simulink library "SUB_ECU_L4_MABX_HW_Interface_PIC_PB"  (R2018a)
settings: Solver=VariableStepAuto  StartTime=0.0  StopTime=10.0  RelTol=1e-3
PostLoadFcn:
  | , if any(exist('dsrtsu_mdlpostloadfcn', 'file') == [2, 3, 6]), try dsrtsu_mdlpostloadfcn('Execute', bdroot); catch fprintf('Error in PostLoadFcn (dsrtsu_mdlpostloadfcn) for model "%s":\n %s\n', bdroot, lasterr); end, end,
undefined symbols (not defined in the file or in its folder): CANR_PROPB_REAX_3_13_CHANNEL_APV, CANR_PROPB_REAX_4_13_CHANNEL_APV, CANR_PROPB_XPR_1_50_CHANNEL_APV, ENUM_CAN_RX_T, ENUM_CAN_TX_T, ENUM_REAX_OPERATION_MODE_T, ENUM_SIGNAL_HEALTH_T, ENUM_XBR_CONTROL_MODE_T, ENUM_XBR_EBI_MODE_T, ENUM_XBR_PASS_THROUGH_ACTIVE_T, ENUM_XBR_PRIORITY_T, ENUM_XPR_INHIBIT_PARK_MANUAL_T, ENUM_XPR_INHIBIT_UNPARK_MANUAL_T, ENUM_XPR_PARK_MANUAL_T, ENUM_XPR_UNPARK_MANUAL_T, PROPB_REAX_1_E4_DES_POS_SIG_SRC_APV, PROPB_REAX_1_E4_DESIRED_OPMODE_APV, PROPB_REAX_1_E4_DESIRED_POSITION_APV, PROPB_REAX_CHANNEL_APV, ptc_matlab_lib
libraries: PTC_MBDS_LIB x293, rtican x158, simulink x61, EmE_MBD_Blockset x38, rti1401lib_dio_type4 x14, simulink_need_slupdate x7, $bdroot x5, rti1401lib_adc_type4 x3, rtmapslib x3, dsa_tcpip_lib x2, SUB_ECU_L4_MABX_HW_Interface_PTC_1571 x1, rtitasklib x1
(part 27 of 49)

== system SUB_ECU_L4_MABX_HW_Interface_PIC_PB/CAN_Out_PIC_PB/CAN_TX_20ms/CAN_TX_STD_ODOMETRY/TX_CAN6 ==
  Enable : Inport
  Data : Inport  Port=2
  Bus Selector4 : BusSelector  OutputSignals=INPUTS.CAN.EBC2_0B.FrontAxleSpeed,INPUTS.CAN.VDC2_0B.SPN1807_SteeringWheelAngle,INPUTS.CAN.VDC2_0B.SPN1808_YawRate,INPUTS.CAN.VDC2_0B.SPN1810_LongitudinalAcceleration
  Data Type Conversion{,1..3} (4 alike) : DataTypeConversion  OutDataTypeStr=double
  Std_OdometryData : rtican/RTICAN Transmit (TX)   Reserved1=[]  Reserved2=[]  Reserved3=[]  Reserved4=[]  SfcnMessage=[]  Msg_Struct=[]  BoardTypeNo=[]  BoardNo=[]  ChannelNo=[]  Parameters=[]  DialogFcn=[]  UnitName=[]  Revision=[]  UnitValues=[]  DSProperties=struct('RTI',struct('Version',uint32(5),'BlockType',struct('isSLSource',uint8(1),'isSLSink',uint8(1),'isHWSource',uint8(0),'isHWSink',uint8(0),'isSetup',uint8(0),'isInline',uint8(1),'isNonInline',uint8(0),'isInterrupt',uint8(0),'isChannelwise',uint8(0)),'IOBoardType','RTICAN','UnitType','MESSAGE','Identifier','TX','DialogType','MSVC','BlockSet','RTICAN','SlaveProcessor','CAN'))  RTIBlockInterface=struct('InputPortsWidth',int32([1 1 1 1]),'InputPortsActive',[1 1 1 1],'InputPortsName',{{'SPN904_FrontAxleSpeed','SPN1807_SteeringWheelAngle','SPN1808_YawRate','SPN1810_LongitudinalAcceleration'}},'InputPortsDataType',{{'SS_DOUBLE','SS_DOUBLE','SS_DOUBLE','SS_DOUBLE'}},'OutputPortsWidth',int32([1 1 1 1]),'OutputPortsActive',[1 1 1 1],'OutputPortsName',{{['TX status'],['TX time'],['TX delta time'],['TX delay time']}},'DialogFcn','rtican_message_interface_gui','BlockDisplay',{{'','center'}},'IconTransparency','on','InitLevel',3,'BlockName',struct('Token',{{'Std_OdometryData'}}),'SampleTime',{{-1}},'TriggerPort',{{'none'}},'EnablePort',{{'yes'}})  RTIBlockParameters="struct('BoardTypeNo',{{1,'OFF',[]}},'BoardNo',{{3,'ON',[1 16]}},'ChannelNo',{{2,'ON',[1 2]}},'Parameters',{{struct('DataFileSupport',struct('DataFileSelectedMaster',1,'DataFileSelectedLocal',0,'DataFileName',['c:\\users\\gavin.coelho\\repos\\l4 svn\\branches\\gennaro\\project_l4\\src\\projectlibrary\\dbc\\mabx_can6_beta4.dbc|c:\\users\\gavin.coelho\\repos\\l4 svn\\branches\\gennaro\\project_l4\\src\\candb\\mabx_can4_chrisbalton.dbc|'],'DataFileDate',{{{['10-Feb-2017 15:17:28']}}},'SelectedFile',['<no file selected>']),'Options',struct('StatusSelected',1,'TimeSelected',1,'DeltaTimeSelected',1,'DelayTimeSelected',1,'DelayTimeTXCommandSelected',0,'EncodeSetUnusedBitsToOne',1,'EnableMsgLoopback',0,'TriggerPort',struct('Selected',0,'TriggerType',0),'EnablePortSelected',1,'SignalOnPortnameSelected',1,'UserCoding',struct('Selected',0,'InterfaceFile','UserEncodingFile','FcnName','UserEncodeFcn','InportSelected',0,'InportWidth',1,'OutportSelected',0,'OutportWidth',1),'TerminationMsg',struct('Selected',0,'Byte0_7','0'),'InitialMsg',struct('Selected',0,'Byte0_7','0')),'Message',struct('MsgOnBlocknameSelected',1,'MsgName','Std_OdometryData','MsgIdFormat',0,'MsgId',10,'MsgLength',8,'NumSignals',4,'SampleTime',-1,'StartTime',struct('Selected',0,'Value',0),'AutoRepeatTime',struct('Selected',0,'Value',0.1),'Timeout',struct('Selected',0,'Value',0.1),'DelayTime',struct('Selected',0,'Value',0.1),'Signal',struct('SgnName',{'SPN904_FrontAxleSpeed','SPN1807_SteeringWheelAngle','SPN1808_YawRate','SPN1810_LongitudinalAcceleration'},'SgnStartBit',{0,16,32,48},'SgnLength',{16,16,16,8},'SgnType',{0,0,0,0},'ModeValue',{-1,-1,-1,-1},'DataType',{0,0,0,0},'ByteLayout',{0,0,0,0},'Factor',{2^-8,2^-10,2^-13,0.1},'Offset',{0,-31.374,-3.92,-12.5},'SgnComment',{{['The average speed of the two front wheels.']},{['The main operator`s steering wheel angle (on the steering column, not the actual wheel angle).']},{['Indicates the rate of rotation about the vertical axis (i.e. the z-axis).  A positive yaw rate signal results when the vehicle turns counter-clockwise.']},{['Indicates the longitudinal acceleration of the vehicle. A positive longitudinal acceleration signal results when the vehicle speed increases, regardless of driving the vehicle forward or backward.']}},'SgnUnit',{'km/h','rad','rad/s','m/s^2'},'Min',{0,0,0,0},'Max',{0,0,0,0},'SLDataType',{'SS_DOUBLE','SS_DOUBLE','SS_DOUBLE','SS_DOUBLE'}),'MsgIdNumFormat',1,'MsgComment',{{''}}),'Version',1.2,'general',struct('isFromLib',0)),'OFF',[]}},'GroupId',{{struct('Group',{{'RTICAN'}},'No',6,'Behavior',{{'NAMECHANGE'}},'BlockType',{{'SINK'}},'NameChangeFlag',0),'OFF',[]}},'SFcnRTICANMessage',{{struct('MsgType','TX','SFcnPortType','Scalar','MsgName','Std_OdometryData','MsgIdFormat','STD','MsgId',10,'MsgLength',8,'NumSignals',4,'SampleTime',-1,'StartTime',struct('Selected','no','Value',0),'AutoRepeatTime',struct('Selected','no','Value',0.1),'Timeout',struct('Selected','no','Value',0.1),'Signal',struct('SgnName',{'SPN904_FrontAxleSpeed','SPN1807_SteeringWheelAngle','SPN1808_YawRate','SPN1810_LongitudinalAcceleration'},'SgnStartBit',{0,16,32,48},'SgnLength',{16,16,16,8},'SgnType',{'standard','standard','standard','standard'},'ModeValue',{-1,-1,-1,-1},'DataType',{['unsigned int'],['unsigned int'],['unsigned int'],['unsigned int']},'ByteLayout',{['little endian'],['little endian'],['little endian'],['little endian']},'Factor',{2^-8,2^-10,2^-13,0.1},'Offset',{0,-31.374,-3.92,-12.5},'SLDataType',{'SS_DOUBLE','SS_DOUBLE','SS_DOUBLE','SS_DOUBLE'}),'StatusSelected','yes','TimeSelected','yes','DeltaTimeSelected','yes','DelayTimeSelected','yes','DelayTimeTXCommandSelected','no','EncodeSetUnusedBitsToOne','yes','EnableMsgLoopback','no','TriggerPort',struct('Selected','no','TriggerType',0),'EnablePortSelected','yes','UserCoding',struct('Selected','no','InterfaceFile','UserEncodingFile','FcnName','UserEncodeFcn','InportSelected','no','InportWidth',1,'OutportSelected','no','OutportWidth',1),'TerminationMsg',struct('Selected','no','Byte0','0x00','Byte1','0x00','Byte2','0x00','Byte3','0x00','Byte4','0x00','Byte5','0x00','Byte6','0x00','Byte7','0x00'),'InitialMsg',struct('Selected','no','Byte0','0x00','Byte1','0x00','Byte2','0x00','Byte3','0x00','Byte4','0x00','Byte5','0x00','Byte6','0x00','Byte7','0x00'),'BoardType','DS1','BoardNo',3,'ControllerNo',2),'OFF',[]}},'TLCFileName',{{'rtican_tx_message','OFF',[]}})"  RTISFcnParameters=struct('SFcnRTICANMessage','struct','TLCFileName','char')  RTIBlockParaDefault=struct('BoardTypeNo',4302,'BoardNo',1,'ChannelNo',1,'Parameters',struct('DataFileSupport',struct('DataFileSelectedMaster',0,'DataFileSelectedLocal',0,'DataFileName','','DataFileDate','','SelectedFile',['<no file selected>']),'Options',struct('StatusSelected',1,'TimeSelected',1,'DeltaTimeSelected',1,'DelayTimeSelected',1,'DelayTimeTXCommandSelected',0,'EncodeSetUnusedBitsToOne',0,'EnableMsgLoopback',0,'TriggerPort',struct('Selected',0,'TriggerType','rising'),'EnablePortSelected',0,'SignalOnPortnameSelected',1,'UserCoding',struct('Selected',0,'InterfaceFile','UserEncodingFile','FcnName','UserEncodeFcn','InportSelected',0,'InportWidth',1,'OutportSelected',0,'OutportWidth',1),'TerminationMsg',struct('Selected',0,'Byte0_7','0'),'InitialMsg',struct('Selected',0,'Byte0_7','0')),'Message',struct('MsgOnBlocknameSelected',0,'MsgName',['TX Message'],'MsgIdFormat',0,'MsgId',100,'MsgLength',8,'NumSignals',1,'SampleTime',-1,'StartTime',struct('Selected',0,'Value',0),'AutoRepeatTime',struct('Selected',0,'Value',0.1),'Timeout',struct('Selected',0,'Value',0.1),'DelayTime',struct('Selected',0,'Value',0.1),'Signal',struct('SgnName',['TX signal'],'SgnStartBit',0,'SgnLength',8,'SgnType',0,'ModeValue',-1,'DataType',0,'SLDataType','SS_DOUBLE','ByteLayout',0,'Factor',1,'Offset',0,'Min',0,'Max',255,'SgnComment',{{}},'SgnUnit',''),'MsgIdNumFormat',0,'MsgComment',{{''}}),'Version',1.2,'general',struct('isFromLib',1)),'GroupId',struct('Group',{{'RTICAN'}},'No',1,'Behavior',{{'NAMECHANGE'}},'BlockType',{{'SINK'}},'NameChangeFlag',0),'SFcnRTICANMessage',struct('MsgType','TX','MsgName',['TX Message'],'MsgIdFormat','STD','MsgId',100,'MsgLength',2,'NumSignals',1,'SampleTime',-1,'StartTime',struct('Selected','no','Value',0),'AutoRepeatTime',struct('Selected','no','Value',0.1),'Timeout',struct('Selected','no','Value',0.1),'DelayTime',struct('Selected','no','Value',0.1),'Signal',struct('SgnName',['TX signal'],'SgnStartBit',0,'SgnLength',8,'SgnType','standard','ModeValue',-1,'DataType',['unsigned int'],'ByteLayout',['little endian'],'SLDataType','SS_DOUBLE','Factor',1,'Offset',0),'StatusSelected','yes','TimeSelected','yes','DeltaTimeSelected','yes','DelayTimeSelected','yes','EnablePortSelected','no','EnableMsgLoopback','no','DelayTimeTXCommandSelected','no','EncodeSetUnusedBitsToOne','no','UserCoding',struct('Selected','no','InterfaceFile','UserDecodingFile','FcnName','UserDecodeFcn','InportSelected','no','InportWidth',1,'OutportSelected','no','OutportWidth',1),'TerminationMsg',struct('Selected','no','Byte0','0x00','Byte1','0x00','Byte2','0x00','Byte3','0x00','Byte4','0x00','Byte5','0x00','Byte6','0x00','Byte7','0x00'),'InitialMsg',struct('Selected','no','Byte0','0x00','Byte1','0x00','Byte2','0x00','Byte3','0x00','Byte4','0x00','Byte5','0x00','Byte6','0x00','Byte7','0x00'),'TriggerPort',struct('Selected','no','TriggerType','rising'),'BoardType','DS4302','BoardNo',1,'ControllerNo',1,'SFcnPortType','Scalar'),'TLCFileName','rtican_tx_message')
      settings: AttributesFormatString=Group Id: RTICAN6\n  SourceProductName=dSPACE RTI CAN Blockset
  Terminator{,1..3} (4 alike) : Terminator
      settings: InitFcn=|
      | try
      |    MBDS_BlockCallback('Update', gcb);
      | end
  wires:
  Data Type Conversion3/1 -> Std_OdometryData/4
  Data Type Conversion2/1 -> Std_OdometryData/3
  Data Type Conversion1/1 -> Std_OdometryData/2
  Data Type Conversion/1 -> Std_OdometryData/1
  Data/1 -> Bus Selector4/1
  Std_OdometryData/1 -> Terminator/1
  Std_OdometryData/3 -> Terminator2/1
  Std_OdometryData/4 -> Terminator3/1
  Std_OdometryData/2 -> Terminator1/1
  Enable/1 -> Std_OdometryData/Enable
  Bus Selector4/3 -> Data Type Conversion2/1  "<SPN1808_YawRate>"
  Bus Selector4/2 -> Data Type Conversion1/1  "<SPN1807_SteeringWheelAngle>"
  Bus Selector4/4 -> Data Type Conversion3/1  "<SPN1810_LongitudinalAcceleration>"
  Bus Selector4/1 -> Data Type Conversion/1  "<FrontAxleSpeed>"

== system SUB_ECU_L4_MABX_HW_Interface_PIC_PB/CAN_Out_PIC_PB/CAN_TX_20ms/Encode_PropB_2C2_XPR/CAN_ID_PropB_2C2_XPR_65 ==
  note: 0xCFF5665
  Bitwise Operator17 : simulink/Logic and Bit Operations/Bitwise Operator  logicop=OR  UseBitMask=off  NumInputPorts=6  BitMask=bin2dec('11011001')  BitMaskRealWorld=Stored Integer
  Data Type Conversion{6..11} (6 alike) : DataTypeConversion  OutDataTypeStr=uint32
  DataPage : Constant  Value=boolean(0)
  ExtendedDataPage : Constant  Value=boolean(0)
  PDUFormat : Constant  Value=uint8(hex2dec('FF'))
  PDUSpecific : Constant  Value=uint8(hex2dec('56'))
  Priority : Constant  Value=uint8(3)
  Shift_Arithmetic 5 : ArithShift  BitShiftNumber=-26
  Shift_Arithmetic 6 : ArithShift  BitShiftNumber=-25
  Shift_Arithmetic 7 : ArithShift  BitShiftNumber=-24
  Shift_Arithmetic 8 : ArithShift  BitShiftNumber=-16
  Shift_Arithmetic 9 : ArithShift  BitShiftNumber=-8
  SourceAddress : Constant  Value=uint8(hex2dec('65'))
  MessageID : Outport
  wires:
  Bitwise Operator17/1 -> MessageID/1
  Data Type Conversion11/1 -> Bitwise Operator17/6
  Data Type Conversion10/1 -> Shift_Arithmetic 9/1
  Data Type Conversion9/1 -> Shift_Arithmetic 8/1
  Data Type Conversion8/1 -> Shift_Arithmetic 7/1
  Data Type Conversion7/1 -> Shift_Arithmetic 6/1
  Data Type Conversion6/1 -> Shift_Arithmetic 5/1
  Shift_Arithmetic 5/1 -> Bitwise Operator17/1
  Shift_Arithmetic 9/1 -> Bitwise Operator17/5
  Shift_Arithmetic 6/1 -> Bitwise Operator17/2
  Shift_Arithmetic 8/1 -> Bitwise Operator17/4
  Shift_Arithmetic 7/1 -> Bitwise Operator17/3
  SourceAddress/1 -> Data Type Conversion11/1
  PDUSpecific/1 -> Data Type Conversion10/1
  PDUFormat/1 -> Data Type Conversion9/1
  DataPage/1 -> Data Type Conversion8/1
  ExtendedDataPage/1 -> Data Type Conversion7/1
  Priority/1 -> Data Type Conversion6/1

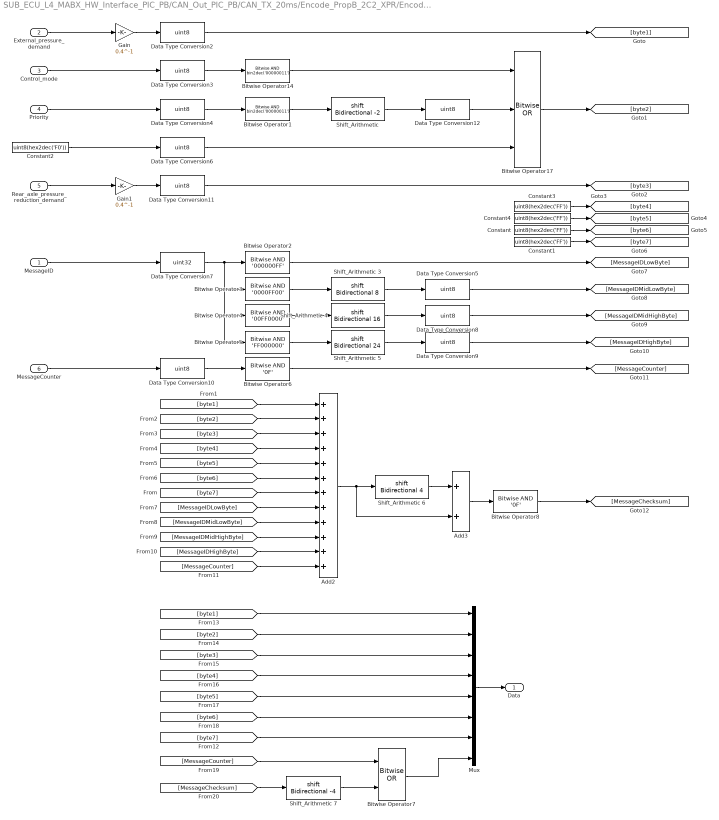
== system SUB_ECU_L4_MABX_HW_Interface_PIC_PB/CAN_Out_PIC_PB/CAN_TX_20ms/Encode_PropB_2C2_XPR/Encode_PropB_2C2_XPR ==
  MessageID : Inport
  External_pressure_demand : Inport  Port=2
  Control_mode : Inport  Port=3
  Priority : Inport  Port=4
  Rear_axle_pressure_reduction_demand : Inport  Port=5
  MessageCounter : Inport  Port=6
  Add2 : Sum  Inputs=++++++++++++  OutDataTypeStr=uint8
  Add3 : Sum  OutDataTypeStr=uint8
  Bitwise Operator1 : simulink/Logic and Bit Operations/Bitwise Operator  logicop=AND  UseBitMask=on  BitMask=bin2dec('00000011')  BitMaskRealWorld=Stored Integer
  Bitwise Operator14 : simulink/Logic and Bit Operations/Bitwise Operator  logicop=AND  UseBitMask=on  BitMask=bin2dec('00000011')  BitMaskRealWorld=Stored Integer
  Bitwise Operator17 : simulink/Logic and Bit Operations/Bitwise Operator  logicop=OR  UseBitMask=off  NumInputPorts=3  BitMask=bin2dec('11011001')  BitMaskRealWorld=Stored Integer
  Bitwise Operator2 : simulink/Logic and Bit Operations/Bitwise Operator  logicop=AND  UseBitMask=on  BitMask='000000FF'  BitMaskRealWorld=Stored Integer
  Bitwise Operator3 : simulink/Logic and Bit Operations/Bitwise Operator  logicop=AND  UseBitMask=on  BitMask='0000FF00'  BitMaskRealWorld=Stored Integer
  Bitwise Operator4 : simulink/Logic and Bit Operations/Bitwise Operator  logicop=AND  UseBitMask=on  BitMask='00FF0000'  BitMaskRealWorld=Stored Integer
  Bitwise Operator5 : simulink/Logic and Bit Operations/Bitwise Operator  logicop=AND  UseBitMask=on  BitMask='FF000000'  BitMaskRealWorld=Stored Integer
  Bitwise Operator6 : simulink/Logic and Bit Operations/Bitwise Operator  logicop=AND  UseBitMask=on  BitMask='0F'  BitMaskRealWorld=Stored Integer
  Bitwise Operator7 : simulink/Logic and Bit Operations/Bitwise Operator  logicop=OR  UseBitMask=off  NumInputPorts=2  BitMask=bin2dec('11011001')  BitMaskRealWorld=Stored Integer
  Bitwise Operator8 : simulink/Logic and Bit Operations/Bitwise Operator  logicop=AND  UseBitMask=on  BitMask='0F'  BitMaskRealWorld=Stored Integer
  Constant{,1,3..4} (4 alike) : Constant  Value=uint8(hex2dec('FF'))
  Constant2 : Constant  Value=uint8(hex2dec('F0'))
  Data Type Conversion{2..6,8..12} (10 alike) : DataTypeConversion  OutDataTypeStr=uint8
  Data Type Conversion7 : DataTypeConversion  OutDataTypeStr=uint32
  Gain : Gain  Gain=0.4^-1
  Gain1 : Gain  Gain=0.4^-1
  Mux : Mux  Inputs=8
  "Shift_Arithmetic " : ArithShift  BitShiftNumber=-2
  Shift_Arithmetic 3 : ArithShift  BitShiftNumber=8
  Shift_Arithmetic 4 : ArithShift  BitShiftNumber=16
  Shift_Arithmetic 5 : ArithShift  BitShiftNumber=24
  Shift_Arithmetic 6 : ArithShift  BitShiftNumber=4
  Shift_Arithmetic 7 : ArithShift  BitShiftNumber=-4
  Data : Outport
  wires:
  [byte7] -> Mux/7
  [byte6] -> Mux/6
  [byte5] -> Mux/5
  [byte4] -> Mux/4
  [byte3] -> Mux/3
  [byte2] -> Mux/2
  [byte1] -> Mux/1
  [byte7] -> Add2/7
  [byte6] -> Add2/6
  [byte5] -> Add2/5
  [byte4] -> Add2/4
  [byte3] -> Add2/3
  [byte2] -> Add2/2
  [byte1] -> Add2/1
  Data Type Conversion6/1 -> Bitwise Operator17/3
  Bitwise Operator17/1 -> [byte2]
  Bitwise Operator1/1 -> "Shift_Arithmetic "/1
  Data Type Conversion3/1 -> Bitwise Operator14/1
  "Shift_Arithmetic "/1 -> Data Type Conversion12/1
  Data Type Conversion4/1 -> Bitwise Operator1/1
  Constant2/1 -> Data Type Conversion6/1
  Bitwise Operator14/1 -> Bitwise Operator17/1
  Data Type Conversion12/1 -> Bitwise Operator17/2
  Data Type Conversion11/1 -> [byte3]
  Rear_axle_pressure_reduction_demand/1 -> Gain1/1
  Constant4/1 -> [byte5]
  Constant3/1 -> [byte4]
  Priority/1 -> Data Type Conversion4/1
  Data Type Conversion7/1 -> Bitwise Operator5/1, Bitwise Operator4/1, Bitwise Operator3/1, Bitwise Operator2/1
  Data Type Conversion10/1 -> Bitwise Operator6/1
  External_pressure_demand/1 -> Gain/1
  Mux/1 -> Data/1
  Bitwise Operator7/1 -> Mux/8
  Shift_Arithmetic 7/1 -> Bitwise Operator7/2
  [MessageChecksum] -> Shift_Arithmetic 7/1
  [MessageCounter] -> Bitwise Operator7/1
  Bitwise Operator8/1 -> [MessageChecksum]
  Add3/1 -> Bitwise Operator8/1
  Shift_Arithmetic 6/1 -> Add3/1
  [MessageIDHighByte] -> Add2/11
  [MessageIDLowByte] -> Add2/8
  [MessageCounter] -> Add2/12
  [MessageIDMidLowByte] -> Add2/9
  [MessageIDMidHighByte] -> Add2/10
  Bitwise Operator6/1 -> [MessageCounter]
  Data Type Conversion9/1 -> [MessageIDHighByte]
  Data Type Conversion8/1 -> [MessageIDMidHighByte]
  Data Type Conversion5/1 -> [MessageIDMidLowByte]
  Bitwise Operator2/1 -> [MessageIDLowByte]
  MessageCounter/1 -> Data Type Conversion10/1
  Shift_Arithmetic 5/1 -> Data Type Conversion9/1
  Shift_Arithmetic 4/1 -> Data Type Conversion8/1
  Shift_Arithmetic 3/1 -> Data Type Conversion5/1
  Bitwise Operator5/1 -> Shift_Arithmetic 5/1
  Bitwise Operator4/1 -> Shift_Arithmetic 4/1
  Bitwise Operator3/1 -> Shift_Arithmetic 3/1
  Add2/1 -> Shift_Arithmetic 6/1, Add3/2
  Constant1/1 -> [byte7]
  Constant/1 -> [byte6]
  Control_mode/1 -> Data Type Conversion3/1
  MessageID/1 -> Data Type Conversion7/1
  Data Type Conversion2/1 -> [byte1]
  Gain/1 -> Data Type Conversion2/1
  Gain1/1 -> Data Type Conversion11/1

== system SUB_ECU_L4_MABX_HW_Interface_PIC_PB/CAN_Out_PIC_PB/CAN_TX_20ms/Encode_PropB_2C2_XPR/PropB_2C2_XPR_MessageCounter ==
  Repeating_Sequence_Stair : PTC_MBDS_LIB/Extras/Sources/Repeating_Sequence_Stair  OutValues=uint8([0 1 2 3 4 5 6 7 8 9 10 11 12 13 14 15].')  OutValues_prev=uint8([0 1 2 3 4 5 6 7 8 9 10 11 12 13 14 15].')  PTC_MBDS_BlockVersion=5.41  PTC_BlockType=PTC_MBDS_Repeating_Sequence_Stair
      settings: SourceProductName=PACCAR Technical Center MBDS Library
  MessageCounter : Outport  InitialOutput=0
  wires:
  Repeating_Sequence_Stair/1 -> MessageCounter/1

== system SUB_ECU_L4_MABX_HW_Interface_PIC_PB/CAN_Out_PIC_PB/CAN_TX_5000ms/CAN_TX_RQST_13_E4/TX_CAN5 ==
  Enable : Inport
  RawData : Inport  Port=2
  OperatorEnable : Inport  Port=3
  AND : PTC_MBDS_LIB/MBDS Standard Library/Basic Operations/Logic and Bit Operations/AND  BitwiseMode=off  Inputs=2  UseBitMask=off  BitMask='A7'  OutDataTypeStr=Inherit: Inherit via back propagation  PTC_MBDS_BlockVersion=5.41  PTC_BlockType=PTC_MBDS_AND
      settings: SourceProductName=PACCAR Technical Center MBDS Library
  Data Type Conversion : DataTypeConversion
  Data Type Conversion1 : DataTypeConversion
  Data Type Conversion2 : DataTypeConversion
  Demux : Demux  Outputs=3
  RQST_13_E4 : rtican/RTICAN Transmit (TX)   Reserved1=[]  Reserved2=[]  Reserved3=[]  Reserved4=[]  SfcnMessage=[]  Msg_Struct=[]  BoardTypeNo=[]  BoardNo=[]  ChannelNo=[]  Parameters=[]  DialogFcn=[]  UnitName=[]  Revision=[]  UnitValues=[]  DSProperties=struct('RTI',struct('Version',uint32(5),'BlockType',struct('isSLSource',uint8(1),'isSLSink',uint8(1),'isHWSource',uint8(0),'isHWSink',uint8(0),'isSetup',uint8(0),'isInline',uint8(1),'isNonInline',uint8(0),'isInterrupt',uint8(0),'isChannelwise',uint8(0)),'IOBoardType','RTICAN','UnitType','MESSAGE','Identifier','TX','DialogType','MSVC','BlockSet','RTICAN','SlaveProcessor','CAN'))  RTIBlockInterface=struct('InputPortsWidth',int32([1 1 1]),'InputPortsActive',[1 1 1],'InputPortsName',{{'byte1','byte2','byte3'}},'InputPortsDataType',{{'SS_DOUBLE','SS_DOUBLE','SS_DOUBLE'}},'OutputPortsWidth',int32([1 1 1 1]),'OutputPortsActive',[1 1 1 1],'OutputPortsName',{{['TX status'],['TX time'],['TX delta time'],['TX delay time']}},'DialogFcn','rtican_message_interface_gui','BlockDisplay',{{'','center'}},'IconTransparency','on','InitLevel',3,'BlockName',struct('Token',{{'RQST_13_E4'}}),'SampleTime',{{-1}},'TriggerPort',{{'none'}},'EnablePort',{{'yes'}})  RTIBlockParameters=struct('BoardTypeNo',{{1,'OFF',[]}},'BoardNo',{{3,'ON',[1 16]}},'ChannelNo',{{1,'ON',[1 2]}},'Parameters',{{struct('DataFileSupport',struct('DataFileSelectedMaster',1,'DataFileSelectedLocal',0,'DataFileName',['c:\users\gavin.coelho\repos\l4 svn\branches\gennaro\project_l4\src\projectlibrary\dbc\mabx_can4_chrisbaltonallstandard.dbc|c:\users\gavin.coelho\repos\l4 svn\branches\gennaro\project_l4\src\projectlibrary\dbc\mabx_can4.dbc|'],'DataFileDate',{{{['11-Nov-2016 14:30:51']}}},'SelectedFile',['<no file selected>']),'Options',struct('StatusSelected',1,'TimeSelected',1,'DeltaTimeSelected',1,'DelayTimeSelected',1,'DelayTimeTXCommandSelected',0,'EncodeSetUnusedBitsToOne',0,'EnableMsgLoopback',0,'TriggerPort',struct('Selected',0,'TriggerType',0),'EnablePortSelected',1,'SignalOnPortnameSelected',1,'UserCoding',struct('Selected',0,'InterfaceFile','UserEncodingFile','FcnName','UserEncodeFcn','InportSelected',0,'InportWidth',1,'OutportSelected',0,'OutportWidth',1),'TerminationMsg',struct('Selected',0,'Byte0_7','0'),'InitialMsg',struct('Selected',0,'Byte0_7','0')),'Message',struct('MsgOnBlocknameSelected',1,'MsgName','RQST_13_E4','MsgIdFormat',1,'MsgId',417993700,'MsgLength',8,'NumSignals',3,'SampleTime',-1,'StartTime',struct('Selected',0,'Value',0),'AutoRepeatTime',struct('Selected',0,'Value',0.1),'Timeout',struct('Selected',0,'Value',0.1),'DelayTime',struct('Selected',0,'Value',0.1),'Signal',struct('SgnName',{'byte1','byte2','byte3'},'SgnStartBit',{0,8,16},'SgnLength',{8,8,8},'SgnType',{0,0,0},'ModeValue',{-1,-1,-1},'DataType',{0,0,0},'ByteLayout',{0,0,0},'Factor',{1,1,1},'Offset',{0,0,0},'SgnComment',{{''},{''},{''}},'SgnUnit',{'','',''},'Min',{0,0,0},'Max',{0,0,0},'SLDataType',{'SS_DOUBLE','SS_DOUBLE','SS_DOUBLE'}),'MsgIdNumFormat',1,'MsgComment',{{['Request message 1']}}),'Version',1.2,'general',struct('isFromLib',0)),'OFF',[]}},'GroupId',{{struct('Group',{{'RTICAN'}},'No',5,'Behavior',{{'NAMECHANGE'}},'BlockType',{{'SINK'}},'NameChangeFlag',0),'OFF',[]}},'SFcnRTICANMessage',{{struct('MsgType','TX','SFcnPortType','Scalar','MsgName','RQST_13_E4','MsgIdFormat','XTD','MsgId',417993700,'MsgLength',8,'NumSignals',3,'SampleTime',-1,'StartTime',struct('Selected','no','Value',0),'AutoRepeatTime',struct('Selected','no','Value',0.1),'Timeout',struct('Selected','no','Value',0.1),'Signal',struct('SgnName',{'byte1','byte2','byte3'},'SgnStartBit',{0,8,16},'SgnLength',{8,8,8},'SgnType',{'standard','standard','standard'},'ModeValue',{-1,-1,-1},'DataType',{['unsigned int'],['unsigned int'],['unsigned int']},'ByteLayout',{['little endian'],['little endian'],['little endian']},'Factor',{1,1,1},'Offset',{0,0,0},'SLDataType',{'SS_DOUBLE','SS_DOUBLE','SS_DOUBLE'}),'StatusSelected','yes','TimeSelected','yes','DeltaTimeSelected','yes','DelayTimeSelected','yes','DelayTimeTXCommandSelected','no','EncodeSetUnusedBitsToOne','no','EnableMsgLoopback','no','TriggerPort',struct('Selected','no','TriggerType',0),'EnablePortSelected','yes','UserCoding',struct('Selected','no','InterfaceFile','UserEncodingFile','FcnName','UserEncodeFcn','InportSelected','no','InportWidth',1,'OutportSelected','no','OutportWidth',1),'TerminationMsg',struct('Selected','no','Byte0','0x00','Byte1','0x00','Byte2','0x00','Byte3','0x00','Byte4','0x00','Byte5','0x00','Byte6','0x00','Byte7','0x00'),'InitialMsg',struct('Selected','no','Byte0','0x00','Byte1','0x00','Byte2','0x00','Byte3','0x00','Byte4','0x00','Byte5','0x00','Byte6','0x00','Byte7','0x00'),'BoardType','DS1','BoardNo',3,'ControllerNo',1),'OFF',[]}},'TLCFileName',{{'rtican_tx_message','OFF',[]}})  RTISFcnParameters=struct('SFcnRTICANMessage','struct','TLCFileName','char')  RTIBlockParaDefault=struct('BoardTypeNo',4302,'BoardNo',1,'ChannelNo',1,'Parameters',struct('DataFileSupport',struct('DataFileSelectedMaster',0,'DataFileSelectedLocal',0,'DataFileName','','DataFileDate','','SelectedFile',['<no file selected>']),'Options',struct('StatusSelected',1,'TimeSelected',1,'DeltaTimeSelected',1,'DelayTimeSelected',1,'DelayTimeTXCommandSelected',0,'EncodeSetUnusedBitsToOne',0,'EnableMsgLoopback',0,'TriggerPort',struct('Selected',0,'TriggerType','rising'),'EnablePortSelected',0,'SignalOnPortnameSelected',1,'UserCoding',struct('Selected',0,'InterfaceFile','UserEncodingFile','FcnName','UserEncodeFcn','InportSelected',0,'InportWidth',1,'OutportSelected',0,'OutportWidth',1),'TerminationMsg',struct('Selected',0,'Byte0_7','0'),'InitialMsg',struct('Selected',0,'Byte0_7','0')),'Message',struct('MsgOnBlocknameSelected',0,'MsgName',['TX Message'],'MsgIdFormat',0,'MsgId',100,'MsgLength',8,'NumSignals',1,'SampleTime',-1,'StartTime',struct('Selected',0,'Value',0),'AutoRepeatTime',struct('Selected',0,'Value',0.1),'Timeout',struct('Selected',0,'Value',0.1),'DelayTime',struct('Selected',0,'Value',0.1),'Signal',struct('SgnName',['TX signal'],'SgnStartBit',0,'SgnLength',8,'SgnType',0,'ModeValue',-1,'DataType',0,'SLDataType','SS_DOUBLE','ByteLayout',0,'Factor',1,'Offset',0,'Min',0,'Max',255,'SgnComment',{{}},'SgnUnit',''),'MsgIdNumFormat',0,'MsgComment',{{''}}),'Version',1.2,'general',struct('isFromLib',1)),'GroupId',struct('Group',{{'RTICAN'}},'No',1,'Behavior',{{'NAMECHANGE'}},'BlockType',{{'SINK'}},'NameChangeFlag',0),'SFcnRTICANMessage',struct('MsgType','TX','MsgName',['TX Message'],'MsgIdFormat','STD','MsgId',100,'MsgLength',2,'NumSignals',1,'SampleTime',-1,'StartTime',struct('Selected','no','Value',0),'AutoRepeatTime',struct('Selected','no','Value',0.1),'Timeout',struct('Selected','no','Value',0.1),'DelayTime',struct('Selected','no','Value',0.1),'Signal',struct('SgnName',['TX signal'],'SgnStartBit',0,'SgnLength',8,'SgnType','standard','ModeValue',-1,'DataType',['unsigned int'],'ByteLayout',['little endian'],'SLDataType','SS_DOUBLE','Factor',1,'Offset',0),'StatusSelected','yes','TimeSelected','yes','DeltaTimeSelected','yes','DelayTimeSelected','yes','EnablePortSelected','no','EnableMsgLoopback','no','DelayTimeTXCommandSelected','no','EncodeSetUnusedBitsToOne','no','UserCoding',struct('Selected','no','InterfaceFile','UserDecodingFile','FcnName','UserDecodeFcn','InportSelected','no','InportWidth',1,'OutportSelected','no','OutportWidth',1),'TerminationMsg',struct('Selected','no','Byte0','0x00','Byte1','0x00','Byte2','0x00','Byte3','0x00','Byte4','0x00','Byte5','0x00','Byte6','0x00','Byte7','0x00'),'InitialMsg',struct('Selected','no','Byte0','0x00','Byte1','0x00','Byte2','0x00','Byte3','0x00','Byte4','0x00','Byte5','0x00','Byte6','0x00','Byte7','0x00'),'TriggerPort',struct('Selected','no','TriggerType','rising'),'BoardType','DS4302','BoardNo',1,'ControllerNo',1,'SFcnPortType','Scalar'),'TLCFileName','rtican_tx_message')
      settings: AttributesFormatString=Group Id: RTICAN5\n  SourceProductName=dSPACE RTI CAN Blockset
  Terminator{,1..3} (4 alike) : Terminator
      settings: InitFcn=|
      | try
      |    MBDS_BlockCallback('Update', gcb);
      | end
  wires:
  Data Type Conversion2/1 -> RQST_13_E4/3
  Data Type Conversion1/1 -> RQST_13_E4/2
  Data Type Conversion/1 -> RQST_13_E4/1
  AND/1 -> RQST_13_E4/Enable
  OperatorEnable/1 -> AND/2
  Demux/3 -> Data Type Conversion2/1
  Demux/2 -> Data Type Conversion1/1
  Demux/1 -> Data Type Conversion/1
  RQST_13_E4/1 -> Terminator/1
  RQST_13_E4/3 -> Terminator2/1
  Enable/1 -> AND/1
  RQST_13_E4/4 -> Terminator3/1
  RQST_13_E4/2 -> Terminator1/1
  RawData/1 -> Demux/1

== system SUB_ECU_L4_MABX_HW_Interface_PIC_PB/CAN_Out_PIC_PB/CAN_TX_VariableRate/CAN_TX_Std_SystemTime_01/TX_CAN6 ==
  Enable : Inport
  Data : Inport  Port=2
  AND : PTC_MBDS_LIB/MBDS Standard Library/Basic Operations/Logic and Bit Operations/AND  BitwiseMode=off  Inputs=2  UseBitMask=off  BitMask='A7'  OutDataTypeStr=Inherit: Inherit via back propagation  PTC_MBDS_BlockVersion=5.41  PTC_BlockType=PTC_MBDS_AND
      settings: SourceProductName=PACCAR Technical Center MBDS Library
  Bus Selector : BusSelector  OutputSignals=INPUTS.CAN.SystemTime.RX_status,INPUTS.CAN.SystemTime.SID,INPUTS.CAN.SystemTime.Source,INPUTS.CAN.SystemTime.Date,INPUTS.CAN.SystemTime.Time
  Constant : Constant  Value=0
  Constant1 : Constant
  Std_SystemTime_01 : rtican/RTICAN Transmit (TX)   Reserved1=[]  Reserved2=[]  Reserved3=[]  Reserved4=[]  SfcnMessage=[]  Msg_Struct=[]  BoardTypeNo=[]  BoardNo=[]  ChannelNo=[]  Parameters=[]  DialogFcn=[]  UnitName=[]  Revision=[]  UnitValues=[]  DSProperties=struct('RTI',struct('Version',uint32(5),'BlockType',struct('isSLSource',uint8(1),'isSLSink',uint8(1),'isHWSource',uint8(0),'isHWSink',uint8(0),'isSetup',uint8(0),'isInline',uint8(1),'isNonInline',uint8(0),'isInterrupt',uint8(0),'isChannelwise',uint8(0)),'IOBoardType','RTICAN','UnitType','MESSAGE','Identifier','TX','DialogType','MSVC','BlockSet','RTICAN','SlaveProcessor','CAN'))  RTIBlockInterface=struct('InputPortsWidth',int32([1 1 1 1 1 1]),'InputPortsActive',[1 1 1 1 1 1],'InputPortsName',{{'SID','Source','Date','Time',['Delay TX command'],'Loop-back'}},'InputPortsDataType',{{'SS_DOUBLE','SS_DOUBLE','SS_DOUBLE','SS_DOUBLE','SS_DOUBLE','SS_DOUBLE'}},'OutputPortsWidth',int32([1 1 1 1]),'OutputPortsActive',[1 1 1 1],'OutputPortsName',{{['TX status'],['TX time'],['TX delta time'],['TX delay time']}},'DialogFcn','rtican_message_interface_gui','BlockDisplay',{{'','center'}},'IconTransparency','on','InitLevel',3,'BlockName',struct('Token',{{'Std_SystemTime_01'}}),'SampleTime',{{-1}},'TriggerPort',{{'none'}},'EnablePort',{{'yes'}})  RTIBlockParameters="struct('BoardTypeNo',{{1,'OFF',[]}},'BoardNo',{{3,'ON',[1 16]}},'ChannelNo',{{2,'ON',[1 2]}},'Parameters',{{struct('DataFileSupport',struct('DataFileSelectedMaster',1,'DataFileSelectedLocal',0,'DataFileName',['c:\\users\\gavin.coelho\\repos\\l4 svn\\branches\\gennaro\\project_l4\\src\\projectlibrary\\dbc\\mabx_can6_beta4.dbc|c:\\users\\gavin.coelho\\repos\\l4 svn\\branches\\gennaro\\project_l4\\src\\candb\\mabx_can4_chrisbalton.dbc|'],'DataFileDate',['15-Feb-2018 08:21:11'],'SelectedFile','dbc\\mabx_can6_beta4.dbc','InterfaceFcn','rtican_dbc_file_parser'),'Options',struct('StatusSelected',1,'TimeSelected',1,'DeltaTimeSelected',1,'DelayTimeSelected',1,'DelayTimeTXCommandSelected',1,'EncodeSetUnusedBitsToOne',0,'EnableMsgLoopback',1,'TriggerPort',struct('Selected',0,'TriggerType',0),'EnablePortSelected',1,'SignalOnPortnameSelected',1,'UserCoding',struct('Selected',0,'InterfaceFile','UserEncodingFile','FcnName','UserEncodeFcn','InportSelected',0,'InportWidth',1,'OutportSelected',0,'OutportWidth',1),'TerminationMsg',struct('Selected',0,'Byte0_7','0'),'InitialMsg',struct('Selected',0,'Byte0_7','0')),'Message',struct('MsgOnBlocknameSelected',1,'MsgName','Std_SystemTime_01','MsgIdFormat',0,'MsgId',5,'MsgLength',8,'NumSignals',4,'SampleTime',-1,'StartTime',struct('Selected',0,'Value',0),'AutoRepeatTime',struct('Selected',0,'Value',0.1),'Timeout',struct('Selected',0,'Value',0.1),'DelayTime',struct('Selected',0,'Value',0.1),'Signal',struct('SgnName',{'SID','Source','Date','Time'},'SgnStartBit',{0,8,16,32},'SgnLength',{8,4,16,32},'SgnType',{0,0,0,0},'ModeValue',{-1,-1,-1,-1},'DataType',{0,0,0,0},'ByteLayout',{0,0,0,0},'Factor',{1,1,1,0.0001},'Offset',{0,0,0,0},'SgnComment',{{['An upward counting number used to tie related information together between different PGNs.For example,SID would be used to tie together COG,SOG and RAIM values to a given Pos.255=no valid Pos fix to tie it to.Range 0 to 250 for valid Pos fixes.']},{['0x0 = GPS, ' char(10) '0x1 =GLONASS, ' char(10) '0x2 = WWV or equivalent Radio Station Time Sync, ' char(10) '0x3 = Local Cesium clock, ' char(10) '0x4 = Local Rubidium clock, ' char(10) '0x5 = Local Crystal clock, ' char(10) '0x6 - 0xE = reserved, ' char(10) '0xF = Null']},{['Days since January 1, 1970,   Date is relative to UTC Time.']},{['24 hour clock, 0 =  midnight,  time is in UTC']}},'SgnUnit',{'','','day','sec'},'Min',{0,0,0,0},'Max',{252,15,65532,86401},'SLDataType',{'SS_DOUBLE','SS_DOUBLE','SS_DOUBLE','SS_DOUBLE'}),'MsgIdNumFormat',1,'MsgComment',{{['The purpose of this PGN is twofold:' char(10) '' char(10) '- To provide a regular transmission of UTC time and date' char(10) '- To provide synchronism '],['for measurement data']}}),'Version',1.2,'general',struct('isFromLib',0)),'OFF',[]}},'GroupId',{{struct('Group',{{'RTICAN'}},'No',6,'Behavior',{{'NAMECHANGE'}},'BlockType',{{'SINK'}},'NameChangeFlag',0),'OFF',[]}},'SFcnRTICANMessage',{{struct('MsgType','TX','SFcnPortType','Scalar','MsgName','Std_SystemTime_01','MsgIdFormat','STD','MsgId',5,'MsgLength',8,'NumSignals',4,'SampleTime',-1,'StartTime',struct('Selected','no','Value',0),'AutoRepeatTime',struct('Selected','no','Value',0.1),'Timeout',struct('Selected','no','Value',0.1),'Signal',struct('SgnName',{'SID','Source','Date','Time'},'SgnStartBit',{0,8,16,32},'SgnLength',{8,4,16,32},'SgnType',{'standard','standard','standard','standard'},'ModeValue',{-1,-1,-1,-1},'DataType',{['unsigned int'],['unsigned int'],['unsigned int'],['unsigned int']},'ByteLayout',{['little endian'],['little endian'],['little endian'],['little endian']},'Factor',{1,1,1,0.0001},'Offset',{0,0,0,0},'SLDataType',{'SS_DOUBLE','SS_DOUBLE','SS_DOUBLE','SS_DOUBLE'}),'StatusSelected','yes','TimeSelected','yes','DeltaTimeSelected','yes','DelayTimeSelected','yes','DelayTimeTXCommandSelected','yes','EncodeSetUnusedBitsToOne','no','EnableMsgLoopback','yes','TriggerPort',struct('Selected','no','TriggerType',0),'EnablePortSelected','yes','UserCoding',struct('Selected','no','InterfaceFile','UserEncodingFile','FcnName','UserEncodeFcn','InportSelected','no','InportWidth',1,'OutportSelected','no','OutportWidth',1),'TerminationMsg',struct('Selected','no','Byte0','0x00','Byte1','0x00','Byte2','0x00','Byte3','0x00','Byte4','0x00','Byte5','0x00','Byte6','0x00','Byte7','0x00'),'InitialMsg',struct('Selected','no','Byte0','0x00','Byte1','0x00','Byte2','0x00','Byte3','0x00','Byte4','0x00','Byte5','0x00','Byte6','0x00','Byte7','0x00'),'BoardType','DS1','BoardNo',3,'ControllerNo',2),'OFF',[]}},'TLCFileName',{{'rtican_tx_message','OFF',[]}})"  RTISFcnParameters=struct('SFcnRTICANMessage','struct','TLCFileName','char')  RTIBlockParaDefault=struct('BoardTypeNo',4302,'BoardNo',1,'ChannelNo',1,'Parameters',struct('DataFileSupport',struct('DataFileSelectedMaster',0,'DataFileSelectedLocal',0,'DataFileName','','DataFileDate','','SelectedFile',['<no file selected>']),'Options',struct('StatusSelected',1,'TimeSelected',1,'DeltaTimeSelected',1,'DelayTimeSelected',1,'DelayTimeTXCommandSelected',0,'EncodeSetUnusedBitsToOne',0,'EnableMsgLoopback',0,'TriggerPort',struct('Selected',0,'TriggerType','rising'),'EnablePortSelected',0,'SignalOnPortnameSelected',1,'UserCoding',struct('Selected',0,'InterfaceFile','UserEncodingFile','FcnName','UserEncodeFcn','InportSelected',0,'InportWidth',1,'OutportSelected',0,'OutportWidth',1),'TerminationMsg',struct('Selected',0,'Byte0_7','0'),'InitialMsg',struct('Selected',0,'Byte0_7','0')),'Message',struct('MsgOnBlocknameSelected',0,'MsgName',['TX Message'],'MsgIdFormat',0,'MsgId',100,'MsgLength',8,'NumSignals',1,'SampleTime',-1,'StartTime',struct('Selected',0,'Value',0),'AutoRepeatTime',struct('Selected',0,'Value',0.1),'Timeout',struct('Selected',0,'Value',0.1),'DelayTime',struct('Selected',0,'Value',0.1),'Signal',struct('SgnName',['TX signal'],'SgnStartBit',0,'SgnLength',8,'SgnType',0,'ModeValue',-1,'DataType',0,'SLDataType','SS_DOUBLE','ByteLayout',0,'Factor',1,'Offset',0,'Min',0,'Max',255,'SgnComment',{{}},'SgnUnit',''),'MsgIdNumFormat',0,'MsgComment',{{''}}),'Version',1.2,'general',struct('isFromLib',1)),'GroupId',struct('Group',{{'RTICAN'}},'No',1,'Behavior',{{'NAMECHANGE'}},'BlockType',{{'SINK'}},'NameChangeFlag',0),'SFcnRTICANMessage',struct('MsgType','TX','MsgName',['TX Message'],'MsgIdFormat','STD','MsgId',100,'MsgLength',2,'NumSignals',1,'SampleTime',-1,'StartTime',struct('Selected','no','Value',0),'AutoRepeatTime',struct('Selected','no','Value',0.1),'Timeout',struct('Selected','no','Value',0.1),'DelayTime',struct('Selected','no','Value',0.1),'Signal',struct('SgnName',['TX signal'],'SgnStartBit',0,'SgnLength',8,'SgnType','standard','ModeValue',-1,'DataType',['unsigned int'],'ByteLayout',['little endian'],'SLDataType','SS_DOUBLE','Factor',1,'Offset',0),'StatusSelected','yes','TimeSelected','yes','DeltaTimeSelected','yes','DelayTimeSelected','yes','EnablePortSelected','no','EnableMsgLoopback','no','DelayTimeTXCommandSelected','no','EncodeSetUnusedBitsToOne','no','UserCoding',struct('Selected','no','InterfaceFile','UserDecodingFile','FcnName','UserDecodeFcn','InportSelected','no','InportWidth',1,'OutportSelected','no','OutportWidth',1),'TerminationMsg',struct('Selected','no','Byte0','0x00','Byte1','0x00','Byte2','0x00','Byte3','0x00','Byte4','0x00','Byte5','0x00','Byte6','0x00','Byte7','0x00'),'InitialMsg',struct('Selected','no','Byte0','0x00','Byte1','0x00','Byte2','0x00','Byte3','0x00','Byte4','0x00','Byte5','0x00','Byte6','0x00','Byte7','0x00'),'TriggerPort',struct('Selected','no','TriggerType','rising'),'BoardType','DS4302','BoardNo',1,'ControllerNo',1,'SFcnPortType','Scalar'),'TLCFileName','rtican_tx_message')
      settings: AttributesFormatString=Group Id: RTICAN6\n  SourceProductName=dSPACE RTI CAN Blockset
  Terminator{,1..3} (4 alike) : Terminator
      settings: InitFcn=|
      | try
      |    MBDS_BlockCallback('Update', gcb);
      | end
  wires:
  Bus Selector/5 -> Std_SystemTime_01/4  "<Time>"
  Bus Selector/4 -> Std_SystemTime_01/3  "<Date>"
  Bus Selector/3 -> Std_SystemTime_01/2  "<Source>"
  Bus Selector/2 -> Std_SystemTime_01/1  "<SID>"
  Data/1 -> Bus Selector/1
  Constant1/1 -> Std_SystemTime_01/6
  Constant/1 -> Std_SystemTime_01/5
  Std_SystemTime_01/2 -> Terminator1/1
  Std_SystemTime_01/4 -> Terminator3/1
  Std_SystemTime_01/3 -> Terminator2/1
  Std_SystemTime_01/1 -> Terminator/1
  Enable/1 -> AND/1
  Bus Selector/1 -> AND/2  "<RX_status>"
  AND/1 -> Std_SystemTime_01/Enable

== system SUB_ECU_L4_MABX_HW_Interface_PIC_PB/CAN_PIC_PB/CAN_RX_EC1_00/CAN_RX_EC1_00/Decode ==
  Inport : Inport
  timeStamp : Inport  Port=2
  Enable : EnablePort
  Selector : Selector  InputPortWidth=39  IndexOptions=Index vector (dialog)  Indices=1:39  OutputSizes=1
  Subtract : Sum  Inputs=+-  OutDataTypeStr=single  SaturateOnIntegerOverflow=on  InputSameDT=on
      settings: AttributesFormatString=Saturate: %<SaturateOnIntegerOverflow>
  Unit_Delay : UnitDelay  SampleTime=-1
      settings: AttributesFormatString=Init = %<InitialCondition>
  RawData : Outport
  RX_time : Outport  Port=2
  RX_delta_time : Outport  Port=3
  wires:
  timeStamp/1 -> Unit_Delay/1, Subtract/1, RX_time/1
  Unit_Delay/1 -> Subtract/2
  Subtract/1 -> RX_delta_time/1
  Inport/1 -> Selector/1
  Selector/1 -> RawData/1

== system SUB_ECU_L4_MABX_HW_Interface_PIC_PB/CAN_PIC_PB/CAN_RX_VI_00/CAN_RX_VI_00/Decode ==
  Inport : Inport
  timeStamp : Inport  Port=2
  Enable : EnablePort
  Selector : Selector  InputPortWidth=17  IndexOptions=Index vector (dialog)  Indices=1:17  OutputSizes=1
  Subtract : Sum  Inputs=+-  OutDataTypeStr=single  SaturateOnIntegerOverflow=on  InputSameDT=on
      settings: AttributesFormatString=Saturate: %<SaturateOnIntegerOverflow>
  Unit_Delay : UnitDelay  SampleTime=-1
      settings: AttributesFormatString=Init = %<InitialCondition>
  RawData : Outport
  RX_time : Outport  Port=2
  RX_delta_time : Outport  Port=3
  wires:
  Selector/1 -> RawData/1
  Inport/1 -> Selector/1
  Subtract/1 -> RX_delta_time/1
  Unit_Delay/1 -> Subtract/2
  timeStamp/1 -> RX_time/1, Subtract/1, Unit_Delay/1

== system SUB_ECU_L4_MABX_HW_Interface_PIC_PB/DIGITAL/PWM pedal input management/Diagnose pedal input signals/Leaky_bucket ==
  Signal_valid_range_max : Inport
  Signal_valid_range_min : Inport  Port=2
  Count_Max : Inport  Port=3
  Count_Min : Inport  Port=4
  Input_signal : Inport  Port=5
  Check Dynamic Range1 : simulink/Model Verification/Check  Dynamic Range  Description=min < u < max  enabled=on  stopWhenAssertionFail=off  export=on  icon=graphic
      settings: SourceProductName=Simulink  SourceProductBaseCode=SL
  Decrement Real World3 : simulink/Additional Math & Discrete/Additional Math: Increment - Decrement/Decrement Real World
      settings: SourceProductName=Simulink  SourceProductBaseCode=SL
  Dynamic_saturation3 : EmE_MBD_Blockset/Discontinuities/Dynamic_saturation
      settings: SourceProductName=PACCAR EmE MBD Blockset
  If_Then_Else3 : EmE_MBD_Blockset/Signal Routing/If_Then_Else
      settings: SourceProductName=PACCAR EmE MBD Blockset
  Increment Real World3 : simulink/Additional Math & Discrete/Additional Math: Increment - Decrement/Increment Real World
      settings: SourceProductName=Simulink  SourceProductBaseCode=SL
  Relational Operator8 : RelationalOperator  Operator=<=  OutDataTypeStr=boolean  RndMeth=Nearest
  Relational Operator9 : RelationalOperator  Operator=~=  OutDataTypeStr=boolean  RndMeth=Nearest
  Unit Delay External IC3 : simulink_need_slupdate/Unit Delay External IC  tsamp=-1
      settings: SourceProductName=Simulink  SourceProductBaseCode=SL
  Fault_Count : Outport
  F_Fault_Soft : Outport  Port=2
  F_Fault_Hard : Outport  Port=3
  wires:
  Count_Min/1 -> Unit Delay External IC3/2, Relational Operator9/2, Dynamic_saturation3/3
  Dynamic_saturation3/1 -> Relational Operator9/1, Unit Delay External IC3/1, Fault_Count/1, Relational Operator8/2  "Fault_Count"
  Decrement Real World3/1 -> If_Then_Else3/2
  Increment Real World3/1 -> If_Then_Else3/3
  Relational Operator9/1 -> F_Fault_Soft/1  "F_Fault_Soft"
  Input_signal/1 -> Check Dynamic Range1/3
  Unit Delay External IC3/1 -> Increment Real World3/1, Decrement Real World3/1
  Count_Max/1 -> Relational Operator8/1, Dynamic_saturation3/1
  Relational Operator8/1 -> F_Fault_Hard/1  "F_Fault_Hard"
  Signal_valid_range_max/1 -> Check Dynamic Range1/1
  Check Dynamic Range1/1 -> If_Then_Else3/1  "f_signal_valid"
  Signal_valid_range_min/1 -> Check Dynamic Range1/2
  If_Then_Else3/1 -> Dynamic_saturation3/2

== system SUB_ECU_L4_MABX_HW_Interface_PIC_PB/DIGITAL/PWM pedal input management/Diagnose pedal input signals/Leaky_bucket1 ==
  Signal_valid_range_max : Inport
  Signal_valid_range_min : Inport  Port=2
  Count_Max : Inport  Port=3
  Count_Min : Inport  Port=4
  Input_signal : Inport  Port=5
  Check Dynamic Range1 : simulink/Model Verification/Check  Dynamic Range  Description=min < u < max  enabled=on  stopWhenAssertionFail=off  export=on  icon=graphic
      settings: SourceProductName=Simulink  SourceProductBaseCode=SL
  Decrement Real World3 : simulink/Additional Math & Discrete/Additional Math: Increment - Decrement/Decrement Real World
      settings: SourceProductName=Simulink  SourceProductBaseCode=SL
  Dynamic_saturation3 : EmE_MBD_Blockset/Discontinuities/Dynamic_saturation
      settings: SourceProductName=PACCAR EmE MBD Blockset
  If_Then_Else3 : EmE_MBD_Blockset/Signal Routing/If_Then_Else
      settings: SourceProductName=PACCAR EmE MBD Blockset
  Increment Real World3 : simulink/Additional Math & Discrete/Additional Math: Increment - Decrement/Increment Real World
      settings: SourceProductName=Simulink  SourceProductBaseCode=SL
  Relational Operator8 : RelationalOperator  Operator=<=  OutDataTypeStr=boolean  RndMeth=Nearest
  Relational Operator9 : RelationalOperator  Operator=~=  OutDataTypeStr=boolean  RndMeth=Nearest
  Unit Delay External IC3 : simulink_need_slupdate/Unit Delay External IC  tsamp=-1
      settings: SourceProductName=Simulink  SourceProductBaseCode=SL
  Fault_Count : Outport
  F_Fault_Soft : Outport  Port=2
  F_Fault_Hard : Outport  Port=3
  wires:
  If_Then_Else3/1 -> Dynamic_saturation3/2
  Signal_valid_range_min/1 -> Check Dynamic Range1/2
  Check Dynamic Range1/1 -> If_Then_Else3/1  "f_signal_valid"
  Signal_valid_range_max/1 -> Check Dynamic Range1/1
  Relational Operator8/1 -> F_Fault_Hard/1  "F_Fault_Hard"
  Count_Max/1 -> Dynamic_saturation3/1, Relational Operator8/1
  Unit Delay External IC3/1 -> Decrement Real World3/1, Increment Real World3/1
  Input_signal/1 -> Check Dynamic Range1/3
  Relational Operator9/1 -> F_Fault_Soft/1  "F_Fault_Soft"
  Increment Real World3/1 -> If_Then_Else3/3
  Decrement Real World3/1 -> If_Then_Else3/2
  Dynamic_saturation3/1 -> Relational Operator8/2, Fault_Count/1, Unit Delay External IC3/1, Relational Operator9/1  "Fault_Count"
  Count_Min/1 -> Dynamic_saturation3/3, Relational Operator9/2, Unit Delay External IC3/2

== system SUB_ECU_L4_MABX_HW_Interface_PIC_PB/DIGITAL/PWM pedal input management/Diagnose pedal input signals/Leaky_bucket2 ==
  Signal_valid_range_max : Inport
  Signal_valid_range_min : Inport  Port=2
  Count_Max : Inport  Port=3
  Count_Min : Inport  Port=4
  Input_signal : Inport  Port=5
  Check Dynamic Range1 : simulink/Model Verification/Check  Dynamic Range  Description=min < u < max  enabled=on  stopWhenAssertionFail=off  export=on  icon=graphic
      settings: SourceProductName=Simulink  SourceProductBaseCode=SL
  Decrement Real World3 : simulink/Additional Math & Discrete/Additional Math: Increment - Decrement/Decrement Real World
      settings: SourceProductName=Simulink  SourceProductBaseCode=SL
  Dynamic_saturation3 : EmE_MBD_Blockset/Discontinuities/Dynamic_saturation
      settings: SourceProductName=PACCAR EmE MBD Blockset
  If_Then_Else3 : EmE_MBD_Blockset/Signal Routing/If_Then_Else
      settings: SourceProductName=PACCAR EmE MBD Blockset
  Increment Real World3 : simulink/Additional Math & Discrete/Additional Math: Increment - Decrement/Increment Real World
      settings: SourceProductName=Simulink  SourceProductBaseCode=SL
  Relational Operator8 : RelationalOperator  Operator=<=  OutDataTypeStr=boolean  RndMeth=Nearest
  Relational Operator9 : RelationalOperator  Operator=~=  OutDataTypeStr=boolean  RndMeth=Nearest
  Unit Delay External IC3 : simulink_need_slupdate/Unit Delay External IC  tsamp=-1
      settings: SourceProductName=Simulink  SourceProductBaseCode=SL
  Fault_Count : Outport
  F_Fault_Soft : Outport  Port=2
  F_Fault_Hard : Outport  Port=3
  wires:
  If_Then_Else3/1 -> Dynamic_saturation3/2
  Signal_valid_range_min/1 -> Check Dynamic Range1/2
  Check Dynamic Range1/1 -> If_Then_Else3/1  "f_signal_valid"
  Signal_valid_range_max/1 -> Check Dynamic Range1/1
  Relational Operator8/1 -> F_Fault_Hard/1  "F_Fault_Hard"
  Count_Max/1 -> Dynamic_saturation3/1, Relational Operator8/1
  Unit Delay External IC3/1 -> Decrement Real World3/1, Increment Real World3/1
  Input_signal/1 -> Check Dynamic Range1/3
  Relational Operator9/1 -> F_Fault_Soft/1  "F_Fault_Soft"
  Increment Real World3/1 -> If_Then_Else3/3
  Decrement Real World3/1 -> If_Then_Else3/2
  Dynamic_saturation3/1 -> Relational Operator8/2, Fault_Count/1, Unit Delay External IC3/1, Relational Operator9/1  "Fault_Count"
  Count_Min/1 -> Dynamic_saturation3/3, Relational Operator9/2, Unit Delay External IC3/2
